simulink model "GeneratorRectifierBoostConverterInverterMotorModel"  (R2021a)
settings: Solver=FixedStepAuto  StartTime=0.0  StopTime=t  FixedStep=tstep  RelTol=1e-3
values from neighbouring files (symbols this model uses):
  boost_catastrophic_fault_toggle = input('   0 = no fault  -or-  1 = fault: ')    [Run_GeneratorRectifierBoostConverterInverterMotorModel.m]    (also in Run_GeneratorRectifierBoostConverterModel.m)
  gen_catastrophic_fault_toggle = input('   0 = no fault  -or-  1 = fault: ')    [Run_GeneratorRectifierBoostConverterInverterMotorModel.m]    (also in Run_GeneratorRectifierBoostConverterModel.m; Run_GeneratorRectifierBuckConverterModel.m; Run_GeneratorRectifierModel.m)
  inv_catastrophic_fault_toggle = input('   0 = no fault  -or-  1 = fault: ')    [Run_GeneratorRectifierBoostConverterInverterMotorModel.m]    (also in Run_InverterMotorModel.m)
  mot_catastrophic_fault_toggle = input('   0 = no fault  -or-  1 = fault: ')    [Run_GeneratorRectifierBoostConverterInverterMotorModel.m]    (also in Run_InverterMotorModel.m)
  rect_catastrophic_fault_toggle = input('   0 = no fault  -or-  1 = fault: ')    [Run_GeneratorRectifierBoostConverterInverterMotorModel.m]    (also in Run_GeneratorRectifierBoostConverterModel.m; Run_GeneratorRectifierBuckConverterModel.m; Run_GeneratorRectifierModel.m)
  tstep = 0.001    [Run_GeneratorRectifierBoostConverterInverterMotorModel.m]    (also in Run_GeneratorRectifierBoostConverterModel.m; Run_GeneratorRectifierBuckConverterModel.m; Run_GeneratorRectifierModel.m; Run_InverterMotorModel.m)
undefined symbols (not defined in the file or in its folder): temp
libraries: PB_Library_Master_Working x5
settings Model: Creator=sfaulk  LastModifiedBy=sfaulk

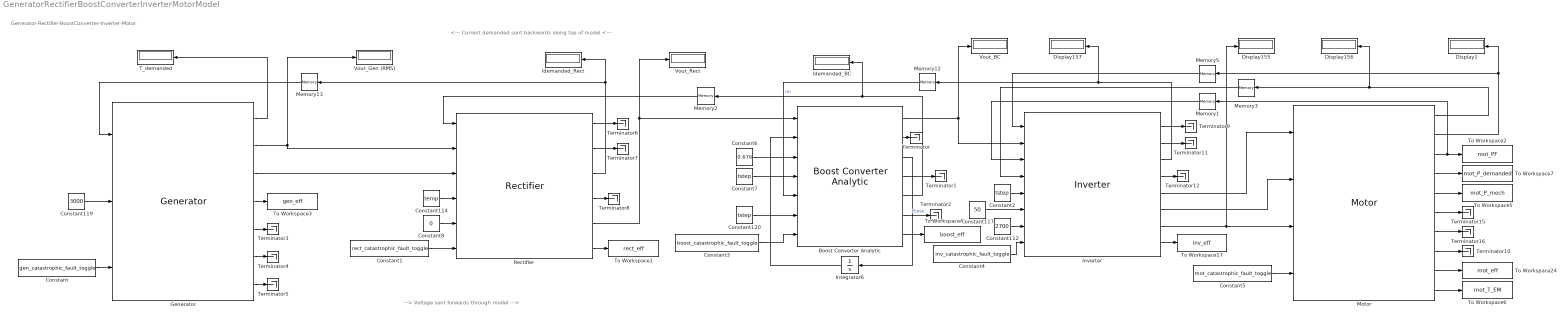
== system GeneratorRectifierBoostConverterInverterMotorModel ==
  note: ---> Voltage sent forwards through model --->
  note: <--- Current demanded sent backwards along top of model <---
  note: Generator-Rectifier-BoostConverter-Inverter-Motor
  Boost Converter Analytic : PB_Library_Master_Working/Boost Converter Analytic  Pdis_M=1  C_M=5e-08  L_M=0.00051  Ron_M=0.784  RC_M=0.26259  RL_M=0.16086  QgTotal_M=4.5e-09  Vdiode_M=0.8  TRise_M=7e-09  TFall_M=2e-09  Fsw_M=250000  Vgate_M=1.7  n_MOSFET=1  MassEst_M=0.37515  TempIn=Celsius  vOut=125  pow=100  minV=47  maxV=53  rippleMode=Use defaults (5% of voltage output and 10% of inductor current)  vRip=.05  iRip=.1  freqMode=Use default frequency (250 kHz)  freq=250e3
      link override "DC - DC Converter/ Dynamic State/State Space Model A1, B1, C1, D1": A_M=[0, 0; 0, -(Ron_M+RL_M)/(L_M*boost_ans.L_M_aDF.Data(end))]  B_M=[0, -1/C_M; 1/(L_M*boost_ans.L_M_aDF.Data(end)), 0]
      link override "DC - DC Converter/ Dynamic State/State Space Model A2, B2, C2, D2": A_M=[0, 1/C_M; -1/(L_M*boost_ans.L_M_aDF.Data(end)), -(Ron_M+RC_M+RL_M)/(L_M*boost_ans.L_M_aDF.Data(end))]  B_M=[0, -1/C_M; 1/(L_M*boost_ans.L_M_aDF.Data(end)), RC_M/(L_M*boost_ans.L_M_aDF.Data(end))]
      link override DC - DC Converter/Constant: Value=[0, 1/C_M; -1/L_M*boost_ans.L_M_aDF.Data(end), -(Ron_M+RC_M+RL_M)/L_M*boost_ans.L_M_aDF.Data(end)]
      link override DC - DC Converter/Steady State/Constant1: Value=[0, 0; 0, -(Ron_M+RL_M)/(L_M*boost_ans.L_M_aDF.Data(end))]
      link override DC - DC Converter/Steady State/Constant2: Value=[0, 1/C_M; -1/(L_M*boost_ans.L_M_aDF.Data(end)), -(Ron_M+RC_M+RL_M)/(L_M*boost_ans.L_M_aDF.Data(end))]
      link override DC - DC Converter/Steady State/Constant3: Value=[0, -1/C_M; 1/(L_M*boost_ans.L_M_aDF.Data(end)), RC_M/(L_M*boost_ans.L_M_aDF.Data(end))]
      link override DC - DC Converter/Steady State/Constant6: Value=[0, -1/C_M; 1/(L_M*boost_ans.L_M_aDF.Data(end)), 0]
      link override DC - DC Converter/Steady State/TemperatureModifiedPerformanceTerm1 /Constant: Value=boost_ans.L_M_aDF.Data(end)
      link override DC - DC Converter/Steady State/TemperatureModifiedPerformanceTerm2 /Constant2: Value=boost_ans.L_M_aDF.Data(end)
      link override DC - DC Converter/Steady State/TemperatureModifiedPerformanceTerm2 /Constant3: Value=boost_ans.L_M_aDF.Data(end)
      link override Power Loss /Constant11: Value=boost_ans.Fsw_M_aDF.Data(end)
      link override Power Loss /Constant12: Value=boost_ans.L_M_aDF.Data(end)
      link override Power Loss /Constant13: Value=boost_ans.Fsw_M_aDF.Data(end)
      link override Power Loss /Constant14: Value=boost_ans.Fsw_M_aDF.Data(end)
      link override Power Loss /Constant15: Value=boost_ans.TFall_M_aDF.Data(end)
      link override Power Loss /Constant7: Value=boost_ans.TRise_M_aDF.Data(end)
  Constant : Constant  Value=gen_catastrophic_fault_toggle
  Constant1 : Constant  Value=rect_catastrophic_fault_toggle
  Constant112 : Constant  Value=2700
  Constant114 : Constant  Value=temp
  Constant117 : Constant  Value=50
  Constant119 : Constant  Value=3000
  Constant120 : Constant  Value=tstep
  Constant2 : Constant  Value=tstep
  Constant3 : Constant  Value=boost_catastrophic_fault_toggle
  Constant4 : Constant  Value=inv_catastrophic_fault_toggle
  Constant5 : Constant  Value=mot_catastrophic_fault_toggle
  Constant6 : Constant  Value=0.676
  Constant7 : Constant  Value=tstep
  Constant8 : Constant  Value=0
  Display{1,155..157} (4 alike) : Display
  Generator : PB_Library_Master_Working/Generator  pp=3  flux_m=0.7  R_s=0.6  L_s=0.02  P_Fe_Nom=900  S_nom=3000  T_nom=70  P_out_max=22000  I_max=36.5  P_in_max=30000  T_max=80  MassEst_M=-1080970  Poles_i=6  R_s_i=.032  L_s_i=.00086+0.00029  S_nom_i=4000  T_nom_i=70  P_out_max_i=22000  I_max_i=36.5  P_in_max_i=30000  K_i=121  V_nom_i=368  T_max_i=80  CalculatePFe=Compute iron losses automatically  P_Fe_Nom_i=0  I_nom_i=36.5  PF_nom_i=0.99  P_Fe_Calc_Flag=1
      link override Constant2: Value=gen_ans.flux_m_aDF.Data(end)
      link override Copper Losses/Constant: Value=gen_ans.R_s_aDF.Data(end)
      link override Copper Losses/Constant1: Value=gen_ans.R_s_aDF.Data(end)
      link override Copper Losses/Degradation Parameter Multiplier/From14: GotoTag=genDI
      link override Copper Losses/Degradation Parameter Multiplier/From15: GotoTag=genDF
      link override Copper Losses/Degradation Parameter Multiplier1/From14: GotoTag=genDI
      link override Copper Losses/Degradation Parameter Multiplier1/From15: GotoTag=genDF
      link override Degradation Input Block/Degradation Input Value: Value=gen_degradation_input
      link override Degradation Parameter Multiplier/From14: GotoTag=genDI
      link override Degradation Parameter Multiplier/From15: GotoTag=genDF
      link override Field Weakening and d current /Constant2: Value=gen_ans.flux_m_aDF.Data(end)
      link override Field Weakening and d current /Degradation Parameter Multiplier/From14: GotoTag=genDI
      link override Field Weakening and d current /Degradation Parameter Multiplier/From15: GotoTag=genDF
      link override Goto4: GotoTag=genDF  TagVisibility=global
      link override Goto6: GotoTag=genDI  TagVisibility=global
      link override Iron Loss/Constant1: Value=gen_ans.P_Fe_Nom_aDF.Data(end)
      link override Iron Loss/Degradation Parameter Multiplier/From14: GotoTag=genDI
      link override Iron Loss/Degradation Parameter Multiplier/From15: GotoTag=genDF
      link override Vdq/Constant: Value=gen_ans.R_s_aDF.Data(end)
      link override Vdq/Constant1: Value=gen_ans.flux_m_aDF.Data(end)
      link override Vdq/Constant2: Value=gen_ans.R_s_aDF.Data(end)
      link override Vdq/Degradation Parameter Multiplier/From14: GotoTag=genDI
      link override Vdq/Degradation Parameter Multiplier/From15: GotoTag=genDF
      link override Vdq/Degradation Parameter Multiplier1/From14: GotoTag=genDI
      link override Vdq/Degradation Parameter Multiplier1/From15: GotoTag=genDF
      link override Vdq/Degradation Parameter Multiplier2/From14: GotoTag=genDI
      link override Vdq/Degradation Parameter Multiplier2/From15: GotoTag=genDF
  Idemanded_BC : Display
  Idemanded_Rect : Display
  Integrator6 : Integrator
  Inverter : PB_Library_Master_Working/Inverter  T_M=[25 175]  u_D_M=[1.16666666666667 0.999999999999998]  u_ce0_M=[0.971428571428571 0.848275862068965]  R_c_M=[0.0285714285714286 0.0551724137931034]  R_D_M=[0.0238095238095238 0.0294117647058824]  E0_M=[6.00000000000002e-05 6.00000000000002e-05]  E1_M=[5.6e-05 5.6e-05]  f_sw_M=20000  L_s_M=0.1  P_max_I=22000  V_phase_I=600  f_sw_I=0  L_s_I=0.1
      link override Diode Conduction Losses/1-D Lookup Table u_D0: Table=u_D_M*inv_ans.u_D_M_aDF.Data(end)
      link override Goto1: GotoTag=FT  TagVisibility=global
      link override Goto2: GotoTag=FT  TagVisibility=global
      link override IGBT Switching Losses/1-D Lookup Table E1: Table=E1_M/inv_ans.E1_M_aDF.Data(end)
      link override IGBT Switching Losses/Constant1: Value=inv_ans.f_sw_M_aDF.Data(end)
      link override IGBT Switching Losses/Degradation Parameter Multiplier/From14: GotoTag=invDI
      link override IGBT Switching Losses/Degradation Parameter Multiplier/From15: GotoTag=invDF
      link override I_Ripple/Constant1: Value=inv_ans.f_sw_M_aDF.Data(end)
      link override I_Ripple/Degradation Parameter Multiplier/From14: GotoTag=invDI
      link override I_Ripple/Degradation Parameter Multiplier/From15: GotoTag=invDF
  Memory{1..3,5,12..13} (6 alike) : Memory
  Motor : PB_Library_Master_Working/Motor  pp=2.5  flux_m=0.7  R_s=0.6  L_s=0.02  P_Fe_Nom=900  S_nom=3000  T_nom=70  P_out_max=22000  I_max=36.5  P_in_max=30000  T_max=80  MassEst_M=-1080970  Poles_i=5  R_s_i=.032  L_s_i=.00086+0.00029  S_nom_i=3000  T_nom_i=70  P_out_max_i=22000  I_max_i=36.5  P_in_max_i=30000  K_i=121  V_nom_i=368  T_max_i=80  CalculatePFe=Compute iron losses automatically  P_Fe_Nom_i=0  I_nom_i=36.5  PF_nom_i=0.99  P_Fe_Calc_Flag=1
      link override Constant8: Value=mot_ans.flux_m_aDF.Data(end)
      link override Copper Losses/Constant: Value=mot_ans.R_s_aDF.Data(end)
      link override Copper Losses/Constant1: Value=mot_ans.R_s_aDF.Data(end)
      link override Copper Losses/Degradation Parameter Multiplier/From14: GotoTag=motDI
      link override Copper Losses/Degradation Parameter Multiplier/From15: GotoTag=motDF
      link override Copper Losses/Degradation Parameter Multiplier1/From14: GotoTag=motDI
      link override Copper Losses/Degradation Parameter Multiplier1/From15: GotoTag=motDF
      link override Degradation Parameter Multiplier/From14: GotoTag=motDI
      link override Degradation Parameter Multiplier/From15: GotoTag=motDF
      link override Field Weakening and d current /Constant2: Value=mot_ans.flux_m_aDF.Data(end)
      link override Field Weakening and d current /Constant3: Value=mot_ans.S_nom_aDF.Data(end)
      link override Field Weakening and d current /Degradation Parameter Multiplier/From14: GotoTag=motDI
      link override Field Weakening and d current /Degradation Parameter Multiplier/From15: GotoTag=motDF
      link override Goto2: TagVisibility=global
      link override Goto3: TagVisibility=global
      link override Iron Loss/Constant1: Value=mot_ans.P_Fe_Nom_aDF.Data(end)
      link override Iron Loss/Constant2: Value=mot_ans.S_nom_aDF.Data(end)
      link override Iron Loss/Degradation Parameter Multiplier/From14: GotoTag=motDI
      link override Iron Loss/Degradation Parameter Multiplier/From15: GotoTag=motDF
      link override Vdq/Constant: Value=mot_ans.flux_m_aDF.Data(end)
      link override Vdq/Constant1: Value=mot_ans.R_s_aDF.Data(end)
      link override Vdq/Constant2: Value=mot_ans.R_s_aDF.Data(end)
      link override Vdq/Degradation Parameter Multiplier/From14: GotoTag=motDI
      link override Vdq/Degradation Parameter Multiplier/From15: GotoTag=motDF
      link override Vdq/Degradation Parameter Multiplier1/From14: GotoTag=motDI
      link override Vdq/Degradation Parameter Multiplier1/From15: GotoTag=motDF
      link override Vdq/Degradation Parameter Multiplier2/From14: GotoTag=motDI
      link override Vdq/Degradation Parameter Multiplier2/From15: GotoTag=motDF
  Rectifier : PB_Library_Master_Working/Rectifier  T_M=[25 175]  u_D_M=[1.16666666666667 0.999999999999998]  u_ce0_M=[0.971428571428571 0.848275862068965]  R_c_M=[0.0285714285714286 0.0551724137931034]  R_D_M=[0.0238095238095238 0.0294117647058824]  E0_M=[6.00000000000002e-05 6.00000000000002e-05]  E1_M=[5.6e-05 5.6e-05]  f_sw_M=20000  L_s_M=0.1  P_max_I=22000  V_phase_I=600  f_sw_I=0  L_s_I=0.1
      link override Degradation Input Block/Degradation Input Value: Value=rect_degradation_input
      link override Diode Conduction Losses1/1-D Lookup Table u_D0: Table=u_D_M/rect_ans.u_D_M_aDF.Data(end)
      link override Goto1: GotoTag=rectDF  TagVisibility=global
      link override Goto2: GotoTag=rectDI  TagVisibility=global
      link override IGBT Switching Losses1/1-D Lookup Table E1: Table=E1_M/inv_ans.E1_M_aDF.Data(end)
      link override IGBT Switching Losses1/Constant1: Value=rect_ans.f_sw_M_aDF.Data(end)
      link override IGBT Switching Losses1/Degradation Parameter Multiplier/From14: GotoTag=rectDI
      link override IGBT Switching Losses1/Degradation Parameter Multiplier/From15: GotoTag=rectDF
      link override I_Ripple1/Constant1: Value=rect_ans.f_sw_M_aDF.Data(end)
      link override I_Ripple1/Degradation Parameter Multiplier/From14: GotoTag=rectDI
      link override I_Ripple1/Degradation Parameter Multiplier/From15: GotoTag=rectDF
  T_demanded : Display
  Terminator{,1..12,15..16} (15 alike) : Terminator
  To Workspace1 : ToWorkspace  VariableName=rect_eff  SaveFormat=Timeseries  SampleTime=-1
  To Workspace17 : ToWorkspace  VariableName=inv_eff  SaveFormat=Timeseries  SampleTime=-1
  To Workspace2 : ToWorkspace  VariableName=mot_PF  SaveFormat=Timeseries  SampleTime=-1
  To Workspace24 : ToWorkspace  VariableName=mot_eff  SaveFormat=Timeseries  SampleTime=-1
  To Workspace3 : ToWorkspace  VariableName=gen_eff  SaveFormat=Timeseries  SampleTime=-1
  To Workspace4 : ToWorkspace  VariableName=boost_eff  SaveFormat=Timeseries  SampleTime=-1
  To Workspace5 : ToWorkspace  VariableName=mot_P_mech  SaveFormat=Timeseries  SampleTime=-1
  To Workspace6 : ToWorkspace  VariableName=mot_T_EM  SaveFormat=Timeseries  SampleTime=-1
  To Workspace7 : ToWorkspace  VariableName=mot_P_demanded  SaveFormat=Timeseries  SampleTime=-1
  Vout_BC : Display
  Vout_Gen (RMS) : Display
  Vout_Rect : Display
  wires:
  Inverter/8 -> To Workspace17/1
  Boost Converter Analytic/3 -> Integrator6/1
  Inverter/3 -> Display157/1, Memory12/1
  Constant4/1 -> Inverter/8
  Rectifier/6 -> To Workspace1/1
  Constant1/1 -> Rectifier/6
  Generator/4 -> To Workspace3/1
  Constant112/1 -> Inverter/7
  Generator/1 -> T_demanded/1
  Boost Converter Analytic/1 -> Inverter/2, Vout_BC/1
  Rectifier/3 -> Memory13/1, Idemanded_Rect/1
  Inverter/5 -> Motor/1
  Constant119/1 -> Generator/2
  Inverter/7 -> Display155/1, Motor/3
  Constant117/1 -> Inverter/6
  Rectifier/5 -> Vout_Rect/1, Boost Converter Analytic/1
  Constant114/1 -> Rectifier/4
  Boost Converter Analytic/5 -> Memory2/1, Idemanded_BC/1  "Iin"
  Constant2/1 -> Inverter/5
  Inverter/6 -> Motor/2
  Memory13/1 -> Generator/1
  Constant5/1 -> Motor/4
  Generator/3 -> Rectifier/3
  Motor/2 -> Memory5/1, Display1/1
  Generator/2 -> Vout_Gen (RMS)/1, Rectifier/2
  Constant/1 -> Generator/3
  Memory12/1 -> Boost Converter Analytic/5
  Constant120/1 -> Boost Converter Analytic/6
  Integrator6/1 -> Boost Converter Analytic/2
  Constant3/1 -> Boost Converter Analytic/7
  Constant6/1 -> Boost Converter Analytic/3
  Constant7/1 -> Boost Converter Analytic/4
  Boost Converter Analytic/2 -> Terminator/1
  Boost Converter Analytic/4 -> Terminator1/1
  Boost Converter Analytic/6 -> Terminator2/1  "PLoss"
  Motor/9 -> To Workspace24/1
  Motor/8 -> Terminator10/1
  Constant8/1 -> Rectifier/5
  Generator/5 -> Terminator3/1
  Generator/7 -> Terminator5/1
  Generator/6 -> Terminator4/1
  Rectifier/1 -> Terminator6/1
  Rectifier/2 -> Terminator7/1
  Rectifier/4 -> Terminator8/1
  Inverter/1 -> Terminator9/1
  Inverter/2 -> Terminator11/1
  Inverter/4 -> Terminator12/1
  Motor/4 -> To Workspace7/1
  Motor/6 -> Terminator15/1
  Motor/7 -> Terminator16/1
  Motor/1 -> Display156/1, Memory3/1
  Memory2/1 -> Rectifier/1
  Memory3/1 -> Inverter/4
  Motor/3 -> To Workspace2/1, Memory1/1
  Memory1/1 -> Inverter/3
  Boost Converter Analytic/7 -> To Workspace4/1
  Memory5/1 -> Inverter/1
  Motor/10 -> To Workspace6/1
  Motor/5 -> To Workspace5/1
